simulink model "simula"  (R2019b)
settings: Solver=VariableStepAuto  StartTime=0.0  StopTime=15  RelTol=1e-3
settings Model: Creator=Claudia Yasar  LastModifiedBy=Claudia Yasar

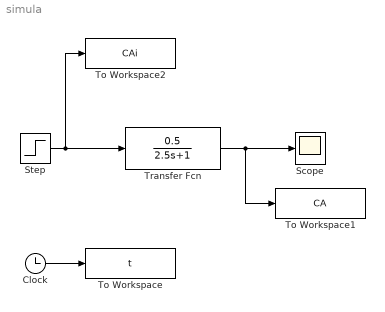
== system simula ==
  Clock : Clock
  Scope : Scope
  Step : Step  Time=0  After=0.3  SampleTime=0
  To Workspace : ToWorkspace  VariableName=t  SampleTime=-1
      settings: Save2DSignal=2-D array (concatenate along first dimension)
  To Workspace1 : ToWorkspace  VariableName=CA  SampleTime=-1
      settings: Save2DSignal=2-D array (concatenate along first dimension)
  To Workspace2 : ToWorkspace  VariableName=CAi  SampleTime=-1
      settings: Save2DSignal=2-D array (concatenate along first dimension)
  Transfer Fcn : TransferFcn  Numerator=[0.5]  Denominator=[2.5 1]
  wires:
  Step/1 -> To Workspace2/1, Transfer Fcn/1
  Transfer Fcn/1 -> To Workspace1/1, Scope/1
  Clock/1 -> To Workspace/1
